simulink model "sheji_3tu"  (Simulink 10.2)
settings: Solver=VariableStepAuto  StartTime=0.0  StopTime=10  RelTol=1e-3
values from neighbouring files (symbols this model uses):
  A = [ 0 1 0 ... (first row only)    [Bujiao_ZuoYe2.m]    (also in fenxi_2.m = [-4 1 0 0 0 0; sheji_1.m = [-1 0 0 0; sheji_1Kong.m = [-1 0 0 0;2 -3 0 0;0 0 2 0;4 -1 2 -4]; sheji_2.m = [-1 0 0 0)
  B = [0 ... (first row only)    [Bujiao_ZuoYe2.m]    (also in fenxi_2.m = [1 3; sheji_1.m = [0;0;1;2]; sheji_1Kong.m = [0;0;1;2]; sheji_2.m = [0;0;1;2])
  C = [0 0 1]    [Bujiao_ZuoYe2.m]    (also in fenxi_2.m = [3 1 0 5 0 0; sheji_1.m = [3 0 1 0]; sheji_1Kong.m = [3 0 1 0]; sheji_2.m = [3 0 1 0])
  G = T*[0;0;G_]    [sheji_2.m]    (also in sheji_3.m; sheji_3Kong.m = T*G2)
  Init = [-0.1 0.1 0.2 -0.3]    [sheji_1.m]    (also in sheji_2.m = [-0.1 0.1 0.2 0.22]; sheji_3.m = [-0.1 0.1 0.2 -0.05]; sheji_3Kong.m)
  Initobserv = [-0.1 0.1 0.1 -0.3]    [sheji_3.m]
  K = [0 0 K_]*T    [sheji_1.m]    (also in sheji_1Kong.m = K2*T; sheji_2.m = place(Ao',Co',P2_); sheji_3.m; sheji_3Kong.m = K2*T)
settings Model: Creator=19017  LastModifiedBy=19017
settings DataIOCC: SaveFormat=Dataset  SignalLoggingSaveFormat=Dataset  ReturnWorkspaceOutputs=on
settings OptimizationCC: LifeSpan=auto
settings DebuggingCC: UnderspecifiedInitializationDetection=Simplified  MergeDetectMultiDrivingBlocksExec=error  FcnCallInpInsideContextMsg=error  SFUnexpectedBacktrackingDiag=error  SFNoUnconditionalDefaultTransitionDiag=error  SFExecutionAtInitializationDiag=warning  ArithmeticOperatorsInVariantConditions=error
settings HardwareCC: ProdBitPerPointer=64  ProdBitPerSizeT=64  ProdBitPerPtrDiffT=64  ProdLargestAtomicFloat=Float  ProdIntDivRoundTo=Zero  ProdEndianess=LittleEndian  ProdWordSize=64  ProdHWDeviceType=Intel->x86-64 (Windows64)
settings ModelReferenceCC: PropagateSignalLabelsOutOfModel=on
settings SFSimCC: SimUseLocalCustomCode=on  CustomCodeUndefinedFunction=FilterOut
settings RTWCC: RTWUseLocalCustomCode=on
settings CodeAppCC: StateflowObjectComments=off
settings GRTTargetCC: TargetLangStandard=C99 (ISO)  CombineOutputUpdateFcns=on  GRTInterface=off
settings ConfigComp: CovMetricSettings=dwe  CovSaveCumulativeToWorkspaceVar=off  CovSaveSingleToWorkspaceVar=off  CovExternalEMLEnable=on

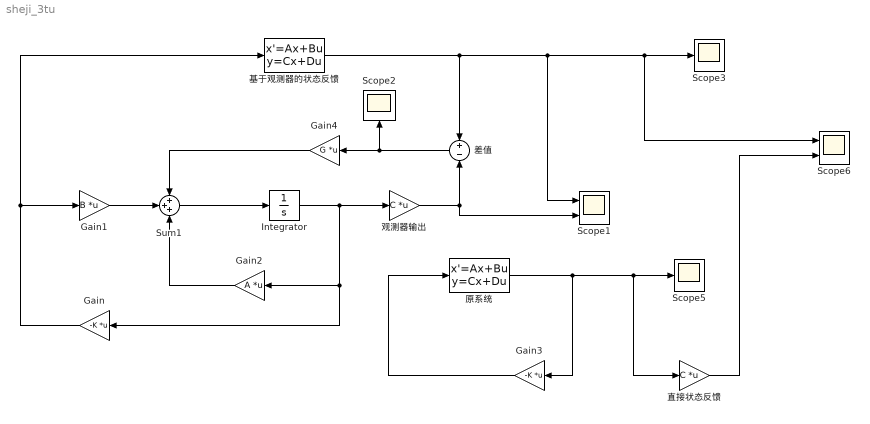
== system sheji_3tu ==
  Gain : Gain  Gain=-K  Multiplication=Matrix(K*u)
  Gain1 : Gain  Gain=B  Multiplication=Matrix(K*u)
  Gain2 : Gain  Gain=A  Multiplication=Matrix(K*u)
  Gain3 : Gain  Gain=-K  Multiplication=Matrix(K*u)
  Gain4 : Gain  Gain=G  Multiplication=Matrix(K*u)
  Integrator : Integrator  InitialCondition=Initobserv
  Scope1 : Scope  NumInputPorts=2
  Scope2 : Scope
  Scope3 : Scope
  Scope5 : Scope
  Scope6 : Scope  NumInputPorts=2
  Sum1 : Sum  Inputs=+++
  原系统 : StateSpace  A=A  B=B  C=eye(4)  D=[0;0;0;0]  InitialCondition=Init
  基于观测器的状态反馈 : StateSpace  A=A  B=B  C=C  D=[0]  InitialCondition=Init
  差值 : Sum  Inputs=+-
  直接状态反馈 : Gain  Gain=C  Multiplication=Matrix(K*u)
  观测器输出 : Gain  Gain=C  Multiplication=Matrix(K*u)
  wires:
  基于观测器的状态反馈/1 -> Scope1/1, Scope6/1, Scope3/1, 差值/1
  差值/1 -> Gain4/1, Scope2/1
  Gain4/1 -> Sum1/1
  Sum1/1 -> Integrator/1
  Integrator/1 -> Gain/1, Gain2/1, 观测器输出/1
  观测器输出/1 -> Scope1/2, 差值/2
  Gain2/1 -> Sum1/3
  Gain1/1 -> Sum1/2
  Gain/1 -> 基于观测器的状态反馈/1, Gain1/1
  原系统/1 -> Gain3/1, 直接状态反馈/1, Scope5/1
  Gain3/1 -> 原系统/1
  直接状态反馈/1 -> Scope6/2
